simulink model "ALFONS_psi_read"  (R2020a)
settings: Solver=FixedStepAuto  StartTime=0.0  StopTime=inf  RelTol=1e-3
libraries: robotlib x2, aerolibanimutils x1
settings Model: Creator=alf  LastModifiedBy=alf
settings OptimizationCC: EnhancedBackFolding=on  PassReuseOutputArgsAs=Individual arguments  ZeroExternalMemoryAtStartup=off  ZeroInternalMemoryAtStartup=off  MaxStackSize=64  OptimizeBlockOrder=speed  DifferentSizesBufferReuse=on  OptimizationCustomize=off  EfficientTunableParamExpr=on
settings DebuggingCC: ParameterTunabilityLossMsg=error
settings HardwareCC: ProdBitPerPointer=32  ProdBitPerSizeT=32  ProdBitPerPtrDiffT=32  ProdLargestAtomicFloat=None  ProdIntDivRoundTo=Undefined  ProdEndianess=Unspecified  ProdWordSize=32  ProdHWDeviceType=Generic->Unspecified (assume 32-bit Generic)
settings SFSimCC: MATLABDynamicMemAlloc=off
settings RTWCC: SystemTargetFile=ert.tlc  HardwareBoard=Robot Operating System (ROS)  TemplateMakefile=ert_default_tmf  Toolchain=Catkin  TargetLang=C++
settings CodeAppCC: ForceParamTrailComments=on  IgnoreCustomStorageClasses=off  OperatorAnnotations=on  SimulinkDataObjDesc=on  SFDataObjDesc=on  InsertBlockDesc=on

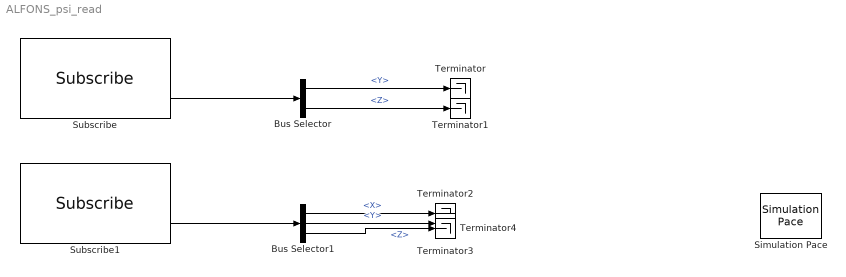
== system ALFONS_psi_read ==
  Bus Selector : BusSelector  OutputSignals=Y,Z
  Bus Selector1 : BusSelector  OutputSignals=X,Y,Z
  Simulation Pace : aerolibanimutils/Simulation Pace  SimulationPace=1  SleepMode=Auto  OutputPaceError=off  SampleTime=1/30
  Subscribe : robotlib/Subscribe  topicSource=Select from ROS network  topic=/psi_ekf_kf  messageType=geometry_msgs/Point  sampleTime=-1  messageQueueLength=1
  Subscribe1 : robotlib/Subscribe  topicSource=Select from ROS network  topic=/psi_ekf  messageType=geometry_msgs/Point  sampleTime=-1  messageQueueLength=1
  Terminator{,1..4} (5 alike) : Terminator
  wires:
  Subscribe/2 -> Bus Selector/1
  Bus Selector/1 -> Terminator/1  "<Y>"
  Bus Selector/2 -> Terminator1/1  "<Z>"
  Subscribe1/2 -> Bus Selector1/1
  Bus Selector1/1 -> Terminator2/1  "<X>"
  Bus Selector1/2 -> Terminator3/1  "<Y>"
  Bus Selector1/3 -> Terminator4/1  "<Z>"
